simulink model "nonlinear_2_tank_model_discrete"  (R2019b)
settings: Solver=VariableStepAuto  StartTime=0.0  StopTime=10.0  RelTol=1e-3
values from neighbouring files (symbols this model uses):
  xe1 = (k_2*sqrt(xe2)/k_1)^2    [script_check_equilibrium_discrete.m]    (also in script_task_2_nonlinear_discrete.m = 1.5563)
  xe2 = 25.53    [script_check_equilibrium_discrete.m]    (also in script_task_2_nonlinear_discrete.m = 4.47)
settings Model: Creator=NicSch02  LastModifiedBy=NicSch02

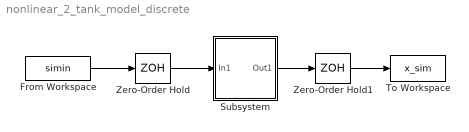
== system nonlinear_2_tank_model_discrete ==
  From Workspace : FromWorkspace  VariableName=simin  SampleTime=0
  Subsystem : Subsystem
  To Workspace : ToWorkspace  VariableName=x_sim  SaveFormat=Structure With Time  SampleTime=-1
  Zero-Order Hold : ZeroOrderHold  SampleTime=-1
  Zero-Order Hold1 : ZeroOrderHold  SampleTime=-1
  wires:
  From Workspace/1 -> Zero-Order Hold/1
  Zero-Order Hold/1 -> Subsystem/1(In1)
  Subsystem/1(Out1) -> Zero-Order Hold1/1
  Zero-Order Hold1/1 -> To Workspace/1

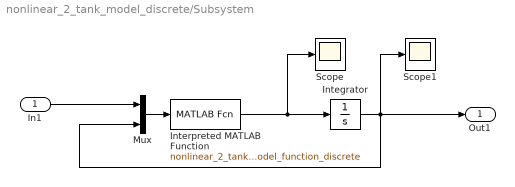
== system nonlinear_2_tank_model_discrete/Subsystem ==
  In1 : Inport
  Integrator : Integrator  InitialCondition=[xe1; xe2;]
  Interpreted MATLAB Function : MATLABFcn  MATLABFcn=nonlinear_2_tank_model_function_discrete
  Mux : Mux  Inputs=2
  Scope : Scope
  Scope1 : Scope
  Out1 : Outport
  wires:
  Mux/1 -> Interpreted MATLAB Function/1
  Integrator/1 -> Out1/1, Scope1/1, Mux/2
  Interpreted MATLAB Function/1 -> Scope/1, Integrator/1
  In1/1 -> Mux/1
